simulink model "Dynamic"  (R2025b)
settings: Solver=FixedStepAuto  StartTime=0.0  StopTime=50  FixedStep=0.01  RelTol=1e-3
libraries: aerolib6dof2 x1
settings Model: DataDictionary=Dynamic_data.sldd  Creator=mauro  LastModifiedBy=mauro

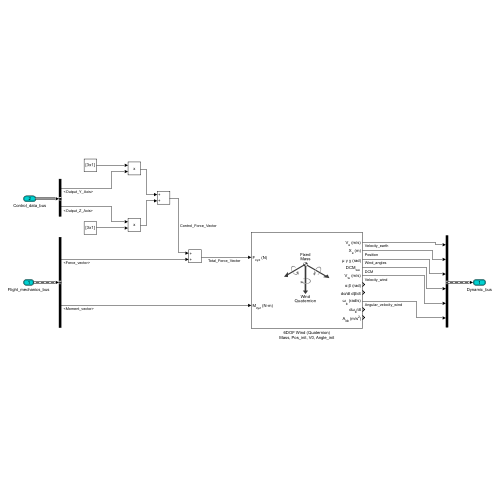
[thumbnail: Simulink's stored preview of the top-level diagram]
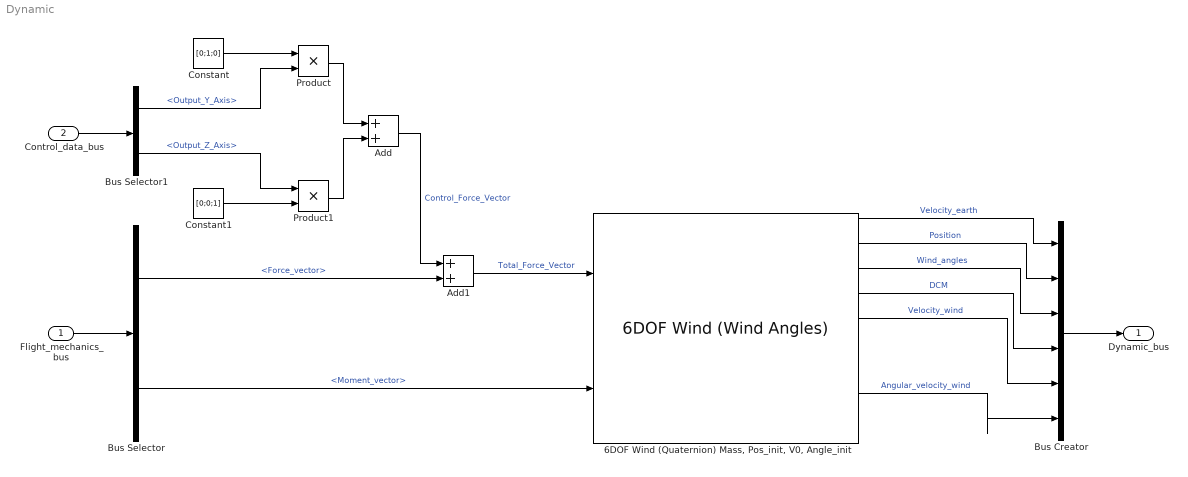
== system Dynamic ==
  Flight_mechanics_bus : Inport  OutDataTypeStr=Bus: Flight_mechanics_bus  BusOutputAsStruct=on
  Control_data_bus : Inport  Port=2  OutDataTypeStr=Bus: Control_data_bus
  "6DOF Wind (Quaternion) Mass, Pos_init, V0, Angle_init" : aerolib6dof2/6DOF Wind (Wind Angles)  units=Metric (MKS)  mtype=Fixed  rep=Quaternion  xme_0=m_pos_init  Vm_0=m_vel_init  wind_0=m_angle_init  pm_0=m_angle_init  mass_0=m_mass  mass_e=0.5  mass_f=2.0  inertia=eye(3)  inertia_e=eye(3)  inertia_f=2*eye(3)  vre_flag=on  abi_flag=off  xme_statename=''  Vm_statename=''  alpha_statename=''  beta_statename=''  wind_statename=''  quat_statename=''  pm_statename=''  mass_statename=''
      settings: LibrarySourceBlock=aerolib6dof2/6DOF Wind (Quaternion)
  Add : Sum
  Add1 : Sum
  Bus Creator : BusCreator  Inputs=6  OutDataTypeStr=Bus: Dynamic_bus  NonVirtualBus=on
  Bus Selector : BusSelector  OutputSignals=Force_vector,Moment_vector
  Bus Selector1 : BusSelector  OutputSignals=Output_Y_Axis,Output_Z_Axis
  Constant : Constant  Value=[0;1;0]
  Constant1 : Constant  Value=[0;0;1]
  Product : Product
  Product1 : Product
  Dynamic_bus : Outport  OutDataTypeStr=Bus: Dynamic_bus  BusOutputAsStruct=on
  wires:
  Flight_mechanics_bus/1 -> Bus Selector/1
  Bus Selector/2 -> "6DOF Wind (Quaternion) Mass, Pos_init, V0, Angle_init"/2  "<Moment_vector>"
  Bus Creator/1 -> Dynamic_bus/1
  "6DOF Wind (Quaternion) Mass, Pos_init, V0, Angle_init"/1 -> Bus Creator/1  "Velocity_earth"
  "6DOF Wind (Quaternion) Mass, Pos_init, V0, Angle_init"/2 -> Bus Creator/2  "Position"
  "6DOF Wind (Quaternion) Mass, Pos_init, V0, Angle_init"/3 -> Bus Creator/3  "Wind_angles"
  "6DOF Wind (Quaternion) Mass, Pos_init, V0, Angle_init"/4 -> Bus Creator/4  "DCM"
  "6DOF Wind (Quaternion) Mass, Pos_init, V0, Angle_init"/5 -> Bus Creator/5  "Velocity_wind"
  "6DOF Wind (Quaternion) Mass, Pos_init, V0, Angle_init"/8 -> Bus Creator/6  "Angular_velocity_wind"
  Bus Selector1/1 -> Product/2  "<Output_Y_Axis>"
  Constant/1 -> Product/1
  Constant1/1 -> Product1/2
  Product/1 -> Add/1
  Add1/1 -> "6DOF Wind (Quaternion) Mass, Pos_init, V0, Angle_init"/1  "Total_Force_Vector"
  Bus Selector/1 -> Add1/2  "<Force_vector>"
  Product1/1 -> Add/2
  Control_data_bus/1 -> Bus Selector1/1
  Add/1 -> Add1/1  "Control_Force_Vector"
  Bus Selector1/2 -> Product1/1  "<Output_Z_Axis>"
